simulink model "Q114"  (R2014b)
settings: Solver=ode45  StartTime=0.0  StopTime=10.0  RelTol=1e-3
settings Model: Creator=asus  LastModifiedBy=Administrator

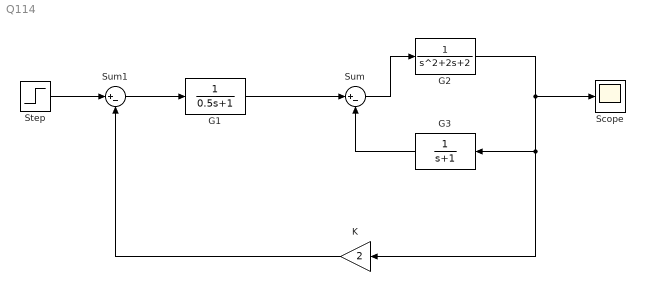
== system Q114 ==
  G1 : TransferFcn  Denominator=[0.5 1]
  G2 : TransferFcn  Denominator=[1 2 2]
  G3 : TransferFcn  Denominator=[1 1]
  K : Gain  Gain=2
  Scope : Scope
  Step : Step  SampleTime=0
  Sum : Sum  Inputs=|+-
  Sum1 : Sum  Inputs=|+-
  wires:
  Sum/1 -> G2/1
  G3/1 -> Sum/2
  G1/1 -> Sum/1
  Sum1/1 -> G1/1
  Step/1 -> Sum1/1
  G2/1 -> K/1, G3/1, Scope/1
  K/1 -> Sum1/2
